simulink model "battery"  (R2018a)
settings: Solver=ode23t  StartTime=0.0  StopTime=15000  RelTol=1e-3
values from neighbouring files (symbols this model uses):
  Initial_SOC = 1    [script_for_battery.m]
  nom_V = 124    [script_for_battery.m]
  normalized_V = [0; 0.35; 0.8; 0.95; 1; 1.02; 1.06; 1.09; 1.12; 1.15; 1.18]    [script_for_battery.m]
  Qmax = 142    [script_for_battery.m]
  SOC = 0:0.1:1    [script_for_battery.m]
libraries: simulink x1
settings Model: Creator=Saurabh Suman  LastModifiedBy=Saurabh Suman

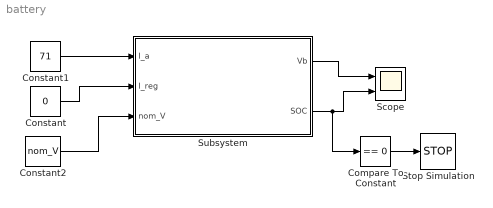
== system battery ==
  Compare To Constant : simulink/Logic and Bit Operations/Compare To Constant  relop===  const=0  OutDataTypeStr=boolean
  Constant : Constant  Value=0
  Constant1 : Constant  Value=71
  Constant2 : Constant  Value=nom_V
  Scope : Scope  NumInputPorts=2
  Stop Simulation : Stop
  Subsystem : Subsystem
  wires:
  Constant1/1 -> Subsystem/1(I_a)
  Constant/1 -> Subsystem/2(I_reg)
  Subsystem/1(Vb) -> Scope/1
  Subsystem/2(SOC) -> Compare To Constant/1, Scope/2
  Compare To Constant/1 -> Stop Simulation/1
  Constant2/1 -> Subsystem/3(nom_V)

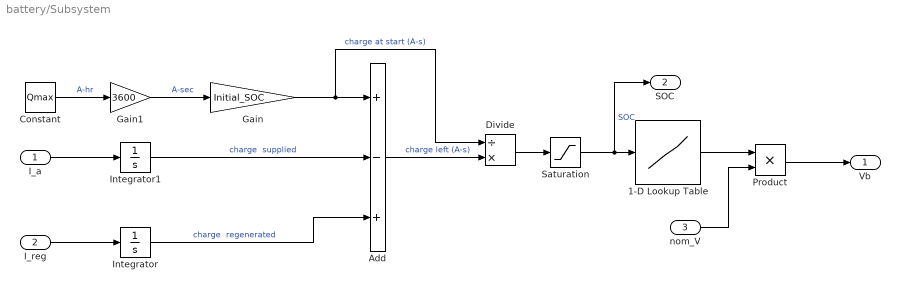
== system battery/Subsystem ==
  I_a : Inport
  I_reg : Inport  Port=2
  nom_V : Inport  Port=3
  1-D Lookup Table : Lookup_n-D  NumberOfTableDimensions=1  BreakpointsForDimension1=SOC  Table=normalized_V  InternalRulePriority=Speed  RndMeth=Simplest  InputSameDT=on
  Add : Sum  Inputs=+-+
  Constant : Constant  Value=Qmax
  Divide : Product  Inputs=/*
  Gain : Gain  Gain=Initial_SOC
  Gain1 : Gain  Gain=3600
  Integrator : Integrator
  Integrator1 : Integrator
  Product : Product
  Saturation : Saturate  UpperLimit=1  LowerLimit=0
  Vb : Outport
  SOC : Outport  Port=2
  wires:
  Add/1 -> Divide/2  "charge left (A-s)"
  Divide/1 -> Saturation/1
  Saturation/1 -> SOC/1, 1-D Lookup Table/1  "SOC"
  I_a/1 -> Integrator1/1
  Gain/1 -> Divide/1, Add/1  "charge at start (A-s)"
  Gain1/1 -> Gain/1  "A-sec"
  Integrator/1 -> Add/3  "charge  regenerated"
  I_reg/1 -> Integrator/1
  Integrator1/1 -> Add/2  "charge  supplied"
  Constant/1 -> Gain1/1  "A-hr"
  Product/1 -> Vb/1
  nom_V/1 -> Product/2
  1-D Lookup Table/1 -> Product/1
